simulink model "san_psk1"  (Simulink 6.5)
settings: Solver=ode45  StartTime=0.0  StopTime=10.0  RelTol=1e-3
libraries: dsparch4 x3, dspsrcs4 x2, simulink_extras x1, commseqgen2 x1
settings Model: Creator=ibm  LastModifiedBy=ibm  BufferReuse=off
settings OptimizationCC: BlockReduction=off  InlineParams=on  BufferReuse=off
settings DebuggingCC: MultiTaskDSMMsg=warning  MultiTaskCondExecSysMsg=none  StrictBusMsg=None
settings RTWCC: IncludeERTFirstTime=on

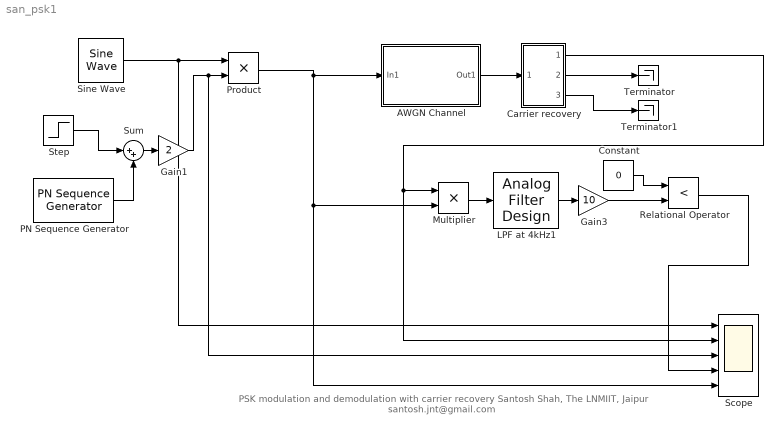
== system san_psk1 ==
  note: PSK modulation and demodulation with carrier recovery
      | Santosh Shah, The LNMIIT, Jaipur
      | santosh.jnt@gmail.com
  AWGN Channel : Subsystem  AncestorBlock=commchan3/AWGN Channel  mask(AWGN Channel){seed=67, noiseMode=Variance from mask, EbNodB=10, EsNodB=10, SNRdB=10, bitsPerSym=100, Ps=1, Tsym=1/300, variance=0.2}
      mask prompts: seed "Initial seed:"; noiseMode "Mode:"; EbNodB "Eb/No (dB):"; EsNodB "Es/No (dB):"; SNRdB "SNR (dB):"; bitsPerSym "Number of bits per symbol:"; Ps "Input signal power (watts):"; Tsym "Symbol period (s):"
      mask help:
      | Add white Gaussian noise to the input signal. The input and output signals can be real or complex. This block supports multichannel input and output signals as well as frame-based processing.
      |
      | When using either of the variance modes with complex inputs, the variance values are equally divided among the real and imaginary components of the input signal.
      mask init:
      | [mode,s]=commblkawgnchan2(gcb,'init');
      | if ~isempty(s.status) error(s.status); end
      mask Help: helpview(commbhelp)
      mask StyleString: edit,popup(Signal to noise ratio  (Eb/No)|Signal to noise ratio  (Es/No)|Signal to noise ratio  (SNR)|Variance from mask|Variance from port),edit,edit,edit,edit,edit,edit,edit
      mask CallbackString: |commblkawgnchan2(gcb,'Mode');|||||||
      mask Display:
      | plot(-10,-10,110, 110,[05 15 10 10 05 10 18 14 13 7.5 13 41 44 47 50 53 57
      | 59 100-[13 7.5 13 14 18 10 5 10 10 15 5]],[70 70 70 85 92 85 79 82 90 88.5
      | 90 90 87 93 87 93 87 90 90 88.5 90 82 79 85 92 85 70 70 70]);
      | disp('AWGN');
      | port_label('input',s.i1,s.i1s);
      | port_label('input',s.i2,s.i2s);
      | port_label('output',s.o1,s.o1s);
  Carrier recovery : Subsystem
  Constant : Constant  Value=0  OutDataType=sfix(16)  ConRadixGroup=Use specified scaling  OutScaling=2^0  SampleTime=inf  FramePeriod=inf
  Gain1 : Gain  Gain=2
  Gain3 : Gain  Gain=10
  LPF at 4kHz1 : dsparch4/Analog Filter Design  method=Butterworth  filttype=Lowpass  N=4  Wlo=4000  Whi=8100  Rp=2  Rs=40
  Multiplier : Product  RndMeth=Zero
  PN Sequence Generator : commseqgen2/PN Sequence Generator  poly=[1 0 0 0 0 1 1]  ini_sta=[0 0 0 0 0 1]  shift=-1  Ts=1/1000  frameBased=off  sampPerFrame=1  reset=off  outDataType=double
  Product : Product  OutDataTypeMode=double  RndMeth=Zero
  Relational Operator : RelationalOperator  Operator=<  LogicOutDataTypeMode=Boolean
  Scope : Scope  NumInputPorts=5
      settings: TimeRange=0.05  YMin=-1~-1~-1~0~-1  YMax=1~1~1~1~1
  Sine Wave : dspsrcs4/Sine Wave  Amplitude=1  Frequency=4000  Phase=0  SampleMode=Discrete  OutComplex=Real  CompMethod=Trigonometric fcn  TableSize=Speed  SampleTime=1/100000  SamplesPerFrame=1  dataType=double  wordLen=16  udDataType=sfix(16)  fracBitsMode=Best precision  numFracBits=15  ResetState=Restart at time zero
  Step : Step  Time=1/300  Before=-.5  After=-.5  SampleTime=0
  Sum : Sum  Inputs=|++
  Terminator : Terminator
  Terminator1 : Terminator
  wires:
  Gain1/1 -> Product/2, Scope/3
  Sum/1 -> Gain1/1
  Step/1 -> Sum/1
  PN Sequence Generator/1 -> Sum/2
  Multiplier/1 -> LPF at 4kHz1/1
  LPF at 4kHz1/1 -> Gain3/1
  Gain3/1 -> Relational Operator/2
  Carrier recovery/1(Out1) -> Multiplier/1, Scope/2
  AWGN Channel/1(Out1) -> Carrier recovery/1(In1)
  Sine Wave/1 -> Product/1, Scope/1
  Carrier recovery/2(Out2) -> Terminator/1
  Carrier recovery/3(Out3) -> Terminator1/1
  Product/1 -> AWGN Channel/1(In1), Multiplier/2, Scope/5
  Constant/1 -> Relational Operator/1
  Relational Operator/1 -> Scope/4

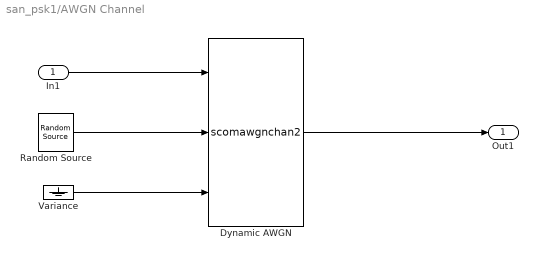
== system san_psk1/AWGN Channel ==
  In1 : Inport
  Dynamic AWGN : S-Function  FunctionName=scomawgnchan2  Parameters=noiseMode, EbNodB, EsNodB, SNRdB, bitsPerSym, Ps, Tsym, variance
  Random Source : dspsrcs4/Random Source  SrcType=Gaussian  NormMethod=Ziggurat  CltLength=12  MinVal=0  MaxVal=1  MeanVal=0  VarVal=1  RepMode=Specify seed  rawSeed=seed  IsInherit=on  SampMode=Discrete  SampTime=1  SampFrame=1  DataType=Double  OutComplex=Real
  Variance : Ground
  Out1 : Outport
  wires:
  Variance/1 -> Dynamic AWGN/3
  Dynamic AWGN/1 -> Out1/1
  In1/1 -> Dynamic AWGN/1
  Random Source/1 -> Dynamic AWGN/2

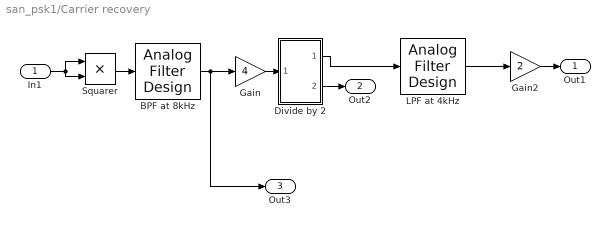
== system san_psk1/Carrier recovery ==
  In1 : Inport
  BPF at 8kHz : dsparch4/Analog Filter Design  method=Butterworth  filttype=Bandpass  N=4  Wlo=7900*2*pi  Whi=8100*2*pi  Rp=2  Rs=40
  Divide by 2 : Subsystem
  Gain : Gain  Gain=4
  Gain2 : Gain  Gain=2
  LPF at 4kHz : dsparch4/Analog Filter Design  method=Butterworth  filttype=Lowpass  N=4  Wlo=4000*2*pi  Whi=4100  Rp=2  Rs=40
  Squarer : Product  RndMeth=Zero
  Out1 : Outport
  Out2 : Outport  Port=2
  Out3 : Outport  Port=3
  wires:
  Squarer/1 -> BPF at 8kHz/1
  BPF at 8kHz/1 -> Gain/1, Out3/1
  LPF at 4kHz/1 -> Gain2/1
  Gain/1 -> Divide by 2/1(Clock)
  Divide by 2/1(Output) -> LPF at 4kHz/1
  In1/1 -> Squarer/1, Squarer/2
  Gain2/1 -> Out1/1
  Divide by 2/2(Output1) -> Out2/1

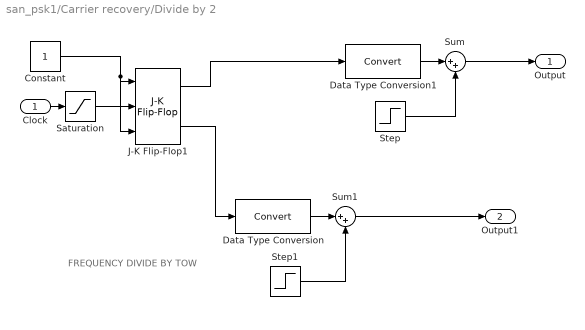
== system san_psk1/Carrier recovery/Divide by 2 ==
  note: FREQUENCY DIVIDE BY TOW
  Clock : Inport
  Constant : Constant  Value=1  OutDataTypeMode=boolean  OutDataType=sfix(16)  ConRadixGroup=Use specified scaling  OutScaling=2^0  SampleTime=inf  FramePeriod=inf
  Data Type Conversion : DataTypeConversion  OutDataTypeMode=double  ConvertRealWorld=Stored Integer (SI)  RndMeth=Nearest
  Data Type Conversion1 : DataTypeConversion  OutDataTypeMode=double  ConvertRealWorld=Stored Integer (SI)  RndMeth=Nearest
  J-K Flip-Flop1 : simulink_extras/Flip Flops/J-K Flip-Flop  SystemSampleTime=-1  initial_condition=0
  Saturation : Saturate  UpperLimit=1  LowerLimit=0
  Step : Step  Time=1/300  Before=-.5  After=-.5  SampleTime=0
  Step1 : Step  Time=1/300  Before=-.5  After=-.5  SampleTime=0
  Sum : Sum  Inputs=|++
  Sum1 : Sum  Inputs=|++
  Output : Outport
  Output1 : Outport  Port=2
  wires:
  J-K Flip-Flop1/1 -> Data Type Conversion1/1
  Constant/1 -> J-K Flip-Flop1/1, J-K Flip-Flop1/3
  J-K Flip-Flop1/2 -> Data Type Conversion/1
  Step1/1 -> Sum1/2
  Data Type Conversion/1 -> Sum1/1
  Sum1/1 -> Output1/1
  Data Type Conversion1/1 -> Sum/1
  Sum/1 -> Output/1
  Step/1 -> Sum/2
  Clock/1 -> Saturation/1
  Saturation/1 -> J-K Flip-Flop1/2
